simulink model "SNS_Deng_CPGDemo"  (R2025a)
settings: Solver=ode1  StartTime=0.0  StopTime=20  FixedStep=1e-4  RelTol=1e-3
libraries: SNS_Library x4
settings Model: Creator=Ben Bolen  LastModifiedBy=Ben Bolen

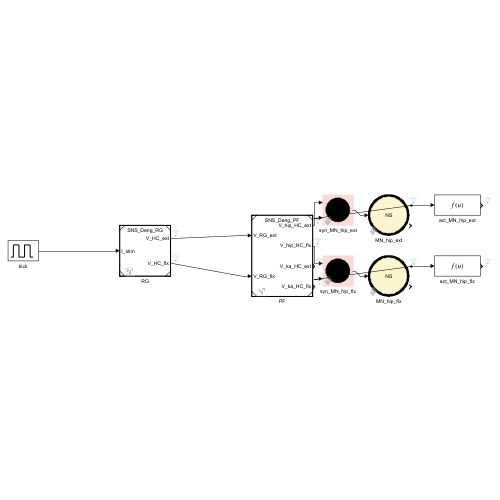
[thumbnail: Simulink's stored preview of the top-level diagram]
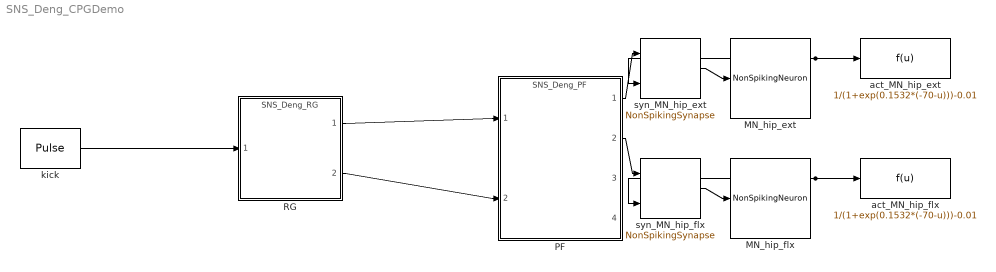
== system SNS_Deng_CPGDemo ==
  MN_hip_ext : SNS_Library/NonSpikingNeuron  Vrest=-100  Gm=1  Cm=5  Thr=-60  Slope=10
  MN_hip_flx : SNS_Library/NonSpikingNeuron  Vrest=-100  Gm=1  Cm=5  Thr=-60  Slope=10
  PF : ModelReference  ModelNameDialog=SNS_Deng_PF.slx  SimulationMode=Normal  ModelReferenceVersion=1.1
  RG : ModelReference  ModelNameDialog=SNS_Deng_RG.slx  SimulationMode=Normal  ModelReferenceVersion=1.1
  act_MN_hip_ext : Fcn  Expr=1/(1+exp(0.1532*(-70-u)))-0.01
  act_MN_hip_flx : Fcn  Expr=1/(1+exp(0.1532*(-70-u)))-0.01
  kick : DiscretePulseGenerator  PulseType=Time based  Amplitude=10  Period=40  PulseWidth=0.05  PhaseDelay=0.1
  syn_MN_hip_ext : SNS_Library/NonSpikingSynapse  gmax=2.565  Esyn=-10  ThrPre=-60  SlopePre=10
  syn_MN_hip_flx : SNS_Library/NonSpikingSynapse  gmax=3.632  Esyn=-10  ThrPre=-60  SlopePre=10
  wires:
  kick/1 -> RG/1
  RG/1 -> PF/1
  RG/2 -> PF/2
  PF/1 -> syn_MN_hip_ext/1
  MN_hip_ext/1 -> syn_MN_hip_ext/2, act_MN_hip_ext/1
  syn_MN_hip_ext/1 -> MN_hip_ext/1
  PF/2 -> syn_MN_hip_flx/1
  MN_hip_flx/1 -> syn_MN_hip_flx/2, act_MN_hip_flx/1
  syn_MN_hip_flx/1 -> MN_hip_flx/1
